simulink model "HeatPump_simplestmodel"  (R2018b)
settings: Solver=VariableStepAuto  StartTime=0.0  StopTime=10000  RelTol=1e-3
values from neighbouring files (symbols this model uses):
  C = 100000    [HeatPump_simplemodel.m]
  cair = 1000    [HeatPump_simplemodel.m]
  cw = 4200    [HeatPump_simplemodel.m]
  Ewp = 1000    [HeatPump_simplemodel.m]
  mc = 0.05    [HeatPump_simplemodel.m]
  me = 0.05    [HeatPump_simplemodel.m]
  Tc_in = 273.15 + 28    (= 301.15)    [HeatPump_simplemodel.m]
  Te_in = 273.15 +7    (= 280.15)    [HeatPump_simplemodel.m]
settings Model: Creator=TrungNguyen  LastModifiedBy=TrungNguyen
settings SFSimCC: SimUseLocalCustomCode=off
settings RTWCC: RTWUseLocalCustomCode=off
settings CodeAppCC: StateflowObjectComments=on

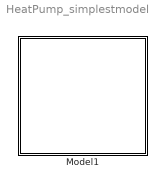
== system HeatPump_simplestmodel ==
  Model1 : Subsystem

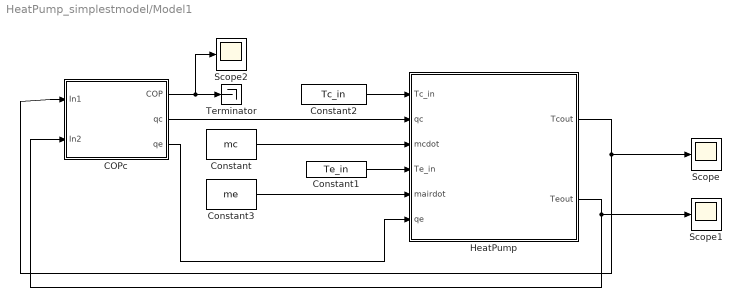
== system HeatPump_simplestmodel/Model1 ==
  COPc : Subsystem
  Constant : Constant  Value=mc
  Constant1 : Constant  Value=Te_in
  Constant2 : Constant  Value=Tc_in
  Constant3 : Constant  Value=me
  HeatPump : Subsystem
  Scope : Scope
  Scope1 : Scope
  Scope2 : Scope
  Terminator : Terminator
  wires:
  COPc/2(qc) -> HeatPump/2(qc)
  HeatPump/1(Tcout) -> Scope/1, COPc/1(In1)
  HeatPump/2(Teout) -> Scope1/1, COPc/2(In2)
  Constant2/1 -> HeatPump/1(Tc_in)
  COPc/3(qe) -> HeatPump/6(qe)
  COPc/1(COP) -> Scope2/1, Terminator/1
  Constant1/1 -> HeatPump/4(Te_in)
  Constant/1 -> HeatPump/3(mcdot)
  Constant3/1 -> HeatPump/5("mairdot ")

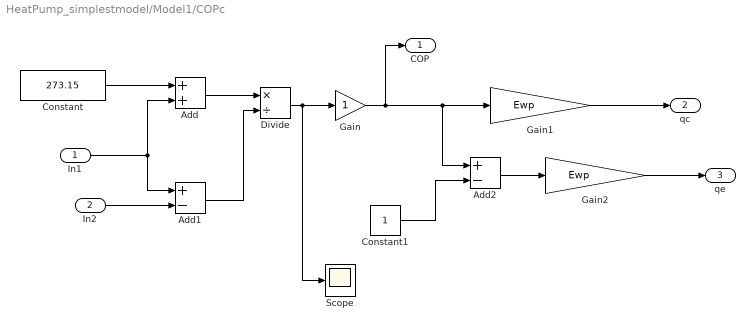
== system HeatPump_simplestmodel/Model1/COPc ==
  In1 : Inport
  In2 : Inport  Port=2
  Add : Sum
  Add1 : Sum  Inputs=+-
  Add2 : Sum  Inputs=+-
  Constant : Constant  Value=273.15
  Constant1 : Constant
  Divide : Product  Inputs=*/
  Gain : Gain
  Gain1 : Gain  Gain=Ewp
  Gain2 : Gain  Gain=Ewp
  Scope : Scope
  COP : Outport
  qc : Outport  Port=2
  qe : Outport  Port=3
  wires:
  Divide/1 -> Scope/1, Gain/1
  In1/1 -> Add1/1, Add/2
  Add1/1 -> Divide/2
  Add/1 -> Divide/1
  Gain/1 -> Add2/1, Gain1/1, COP/1
  Constant/1 -> Add/1
  In2/1 -> Add1/2
  Gain1/1 -> qc/1
  Constant1/1 -> Add2/2
  Add2/1 -> Gain2/1
  Gain2/1 -> qe/1

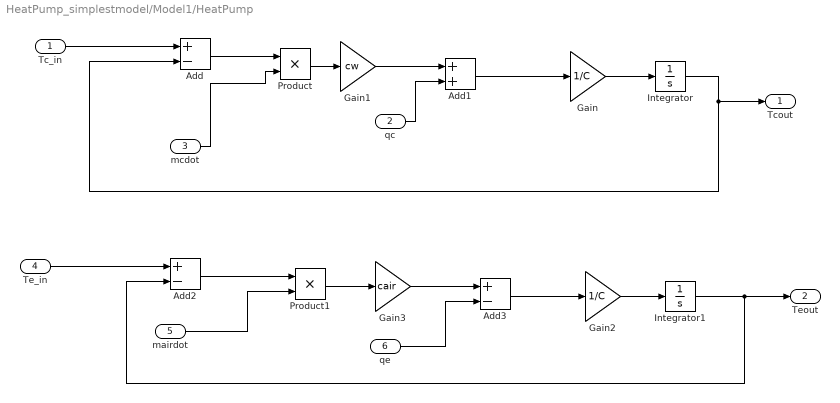
== system HeatPump_simplestmodel/Model1/HeatPump ==
  Tc_in : Inport
  qc : Inport  Port=2
  mcdot : Inport  Port=3
  Te_in : Inport  Port=4
  "mairdot " : Inport  Port=5
  qe : Inport  Port=6
  Add : Sum  Inputs=+-
  Add1 : Sum
  Add2 : Sum  Inputs=+-
  Add3 : Sum  Inputs=+-
  Gain : Gain  Gain=1/C
  Gain1 : Gain  Gain=cw
  Gain2 : Gain  Gain=1/C
  Gain3 : Gain  Gain=cair
  Integrator : Integrator  InitialCondition=26.5+273
  Integrator1 : Integrator  InitialCondition=273
  Product : Product
  Product1 : Product
  Tcout : Outport
  Teout : Outport  Port=2
  wires:
  Product/1 -> Gain1/1
  Add3/1 -> Gain2/1
  qc/1 -> Add1/2
  Add/1 -> Product/1
  "mairdot "/1 -> Product1/2
  Product1/1 -> Gain3/1
  mcdot/1 -> Product/2
  Gain3/1 -> Add3/1
  Add1/1 -> Gain/1
  Tc_in/1 -> Add/1
  qe/1 -> Add3/2
  Gain2/1 -> Integrator1/1
  Add2/1 -> Product1/1
  Integrator1/1 -> Teout/1, Add2/2
  Te_in/1 -> Add2/1
  Integrator/1 -> Tcout/1, Add/2
  Gain1/1 -> Add1/1
  Gain/1 -> Integrator/1
